simulink model "HardThreshold"  (R2020a)
settings: Solver=VariableStepAuto  StartTime=0.0  StopTime=100  RelTol=1e-3
model workspace (MAT data in the model file):
  a = 0
undefined symbols (not defined in the file): fs, th
libraries: simulink x2, dspswit3 x1, dspfdesign x1, hdlsllib x1
settings Model: SimulationMode=rapid-accelerator  Creator=sbuccelli  LastModifiedBy=diflo

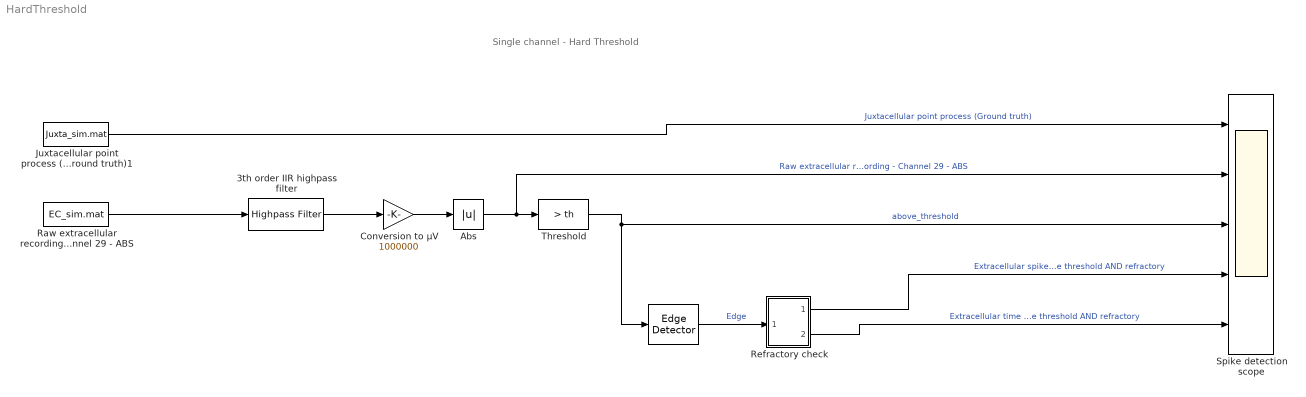
== system HardThreshold ==
  note: Single channel - Hard Threshold
  " " : dspswit3/Edge Detector  InputProcessing=Columns as channels (frame based)
      settings: SourceProductBaseCode=DS
  3th order IIR highpass filter : dspfdesign/Highpass Filter  FilterType=IIR  DesignForMinimumOrder=off  FilterOrder=3  StopbandFrequency=1  PassbandFrequency=300  StopbandAttenuation=80  PassbandRipple=0.1  InheritSampleRate=off  SampleRate=fs  SimulateUsing=Interpreted execution  roundingMode=Floor  coeffsDataTypeStr=fixdt(1,16)
  Abs : Abs
  "Conversion to μV " : Gain  Gain=1000000
  Juxtacellular point process (Ground truth)1 : FromFile  FileName=Juxta_sim.mat  SampleTime=1/fs
  Raw extracellular recording - Channel 29 - ABS : FromFile  FileName=EC_sim.mat  SampleTime=1/fs
  Refractory check : Subsystem
  Spike detection scope : Scope  NumInputPorts=5
  Threshold : simulink/Logic and Bit Operations/Compare To Constant  relop=>  const=th  OutDataTypeStr=boolean
  wires:
  Threshold/1 -> " "/1, Spike detection scope/3  "above_threshold"
  Juxtacellular point process (Ground truth)1/1 -> Spike detection scope/1  "Juxtacellular point process (Ground truth)"
  Raw extracellular recording - Channel 29 - ABS/1 -> 3th order IIR highpass filter/1
  3th order IIR highpass filter/1 -> "Conversion to μV "/1
  "Conversion to μV "/1 -> Abs/1
  " "/1 -> Refractory check/1("   ")  "Edge"
  Refractory check/1(" ") -> Spike detection scope/4  "Extracellular spikes above threshold AND refractory"
  Refractory check/2(Output) -> Spike detection scope/5  "Extracellular time since last spike above threshold AND refractory"
  Abs/1 -> Threshold/1, Spike detection scope/2  "Raw extracellular recording - Channel 29 - ABS"

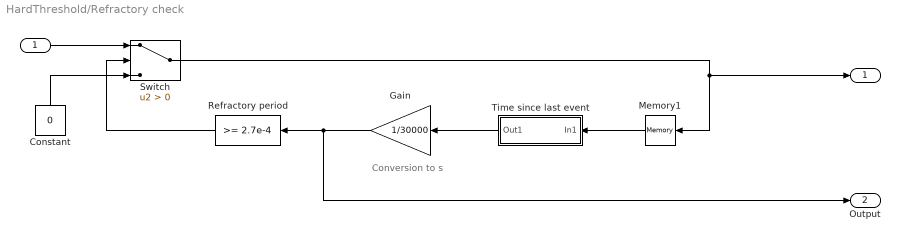
== system HardThreshold/Refractory check ==
  note: Conversion to s
  "   " : Inport
  Constant : Constant  Value=0
  Gain : Gain  Gain=1/30000  ParamDataTypeStr=double
  Memory1 : Memory  InheritSampleTime=on
  Refractory period : simulink/Logic and Bit Operations/Compare To Constant  relop=>=  const=2.7e-4  OutDataTypeStr=boolean
  Switch : Switch  Criteria=u2 > Threshold
  Time since last event : Subsystem
  " " : Outport
  Output : Outport  Port=2
  wires:
  "   "/1 -> Switch/1
  Memory1/1 -> Time since last event/1(In1)
  Time since last event/1(Out1) -> Gain/1
  Constant/1 -> Switch/3
  Gain/1 -> Refractory period/1, Output/1
  Switch/1 -> " "/1, Memory1/1
  Refractory period/1 -> Switch/2

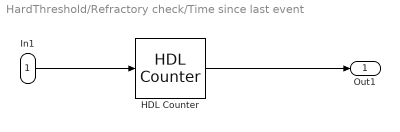
== system HardThreshold/Refractory check/Time since last event ==
  In1 : Inport
  HDL Counter : hdlsllib/Sources/HDL Counter  CountType=Free running  CountInit=1  CountStep=1  CountMax=25  CountFromType=Initial value  CountFrom=1  CountResetPort=on  CountLoadPort=off  CountEnbPort=off  CountDirPort=off  CountDataType=Unsigned  CountWordLen=32  CountFracLen=0  CountSampTime=1
  Out1 : Outport
  wires:
  In1/1 -> HDL Counter/1
  HDL Counter/1 -> Out1/1
